simulink model "missileSystem"  (R2014a)
settings: Solver=ode45  StartTime=0.0  StopTime=10.0  MaxStep=0.2  RelTol=1e-3
values from neighbouring files (symbols this model uses):
  Arb = [A11 A12; A21 A22]    [getRigidBodySS.m]
  Brb = [B1;B2]    [getRigidBodySS.m]
  Crb = [Cx; CAccCG; CAcc]    [getRigidBodySS.m]
  Drb = [Dx; DAccCG; DAcc]    [getRigidBodySS.m]
  wF = 2*pi*50    (= 314.159265359)    [initMissilelFullIO.m]
  wT = 2*pi*25    (= 157.079632679)    [initMissilelFullIO.m]
  zF = 0.707    [initMissilelFullIO.m]
  zT = 0.707    [initMissilelFullIO.m]
libraries: RCTblocks x1
settings Model: Creator=s220385  LastModifiedBy=s220385
settings OptimizationCC: SimCompilerOptimization=off
settings DebuggingCC: MergeDetectMultiDrivingBlocksExec=error  FrameProcessingCompatibilityMsg=error
settings RTWCC: RTWCompilerOptimization=off

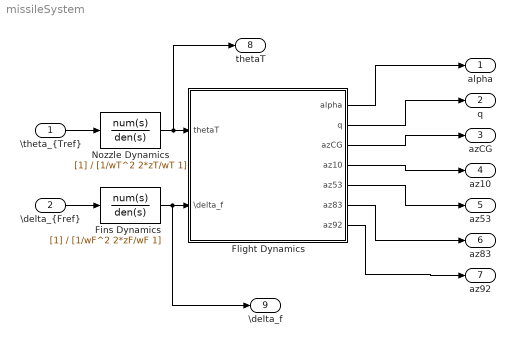
== system missileSystem ==
  "\\theta_{Tref}" : Inport
  "\\delta_{Fref}" : Inport  Port=2
  Fins Dynamics : TransferFcn  Denominator=[1/wF^2 2*zF/wF 1]
  Flight Dynamics : Subsystem  TreatAsAtomicUnit=on
      mask Display:
      | port_label('input', 1, '\theta_T','texmode','on')
      | port_label('input', 2, '\delta_F','texmode','on')
      | 
      | port_label('output', 1, '\alpha','texmode','on')
      | port_label('output', 2, 'q','texmode','on')
      | port_label('output', 3, 'a_{zCG}','texmode','on')
      | port_label('output', 4, 'a_{z10}','texmode','on')
      | port_label('output', 5, 'a_{z53}','texmode','on')
      | port_label('output', 6, 'a_{z83}','texmode','on')
      | port_label('output', 7, 'a_{z91}','texmode','on')
  Nozzle Dynamics : TransferFcn  Denominator=[1/wT^2 2*zT/wT 1]
  alpha : Outport
  q : Outport  Port=2
  azCG : Outport  Port=3
  az10 : Outport  Port=4
  az53 : Outport  Port=5
  az83 : Outport  Port=6
  az92 : Outport  Port=7
  "thetaT " : Outport  Port=8
  \delta_f : Outport  Port=9
  wires:
  Flight Dynamics/4(az10) -> az10/1
  Flight Dynamics/2(q) -> q/1
  Flight Dynamics/1(alpha) -> alpha/1
  "\\theta_{Tref}"/1 -> Nozzle Dynamics/1
  Flight Dynamics/3(azCG) -> azCG/1
  Flight Dynamics/5(az53) -> az53/1
  Flight Dynamics/6(az83) -> az83/1
  Flight Dynamics/7(az92) -> az92/1
  Nozzle Dynamics/1 -> "thetaT "/1, Flight Dynamics/1(thetaT)
  Fins Dynamics/1 -> \delta_f/1, Flight Dynamics/2(\delta_f)
  "\\delta_{Fref}"/1 -> Fins Dynamics/1

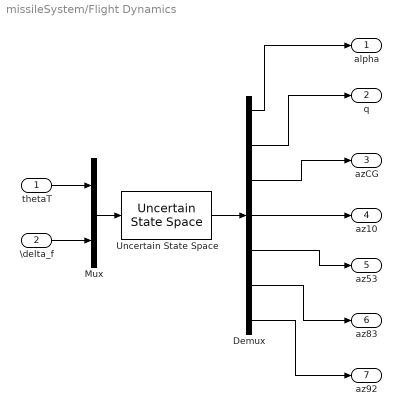
== system missileSystem/Flight Dynamics ==
  thetaT : Inport
  \delta_f : Inport  Port=2
  Demux : Demux  Outputs=7
  Mux : Mux  Inputs=2
  Uncertain State Space : RCTblocks/Uncertain State Space  Tag=USS  USystem=ss(Arb,Brb,Crb,Drb)  UValue=[]  X0=[]  uX0=[]
  alpha : Outport
  q : Outport  Port=2
  azCG : Outport  Port=3
  az10 : Outport  Port=4
  az53 : Outport  Port=5
  az83 : Outport  Port=6
  az92 : Outport  Port=7
  wires:
  Demux/3 -> azCG/1
  Demux/2 -> q/1
  Demux/4 -> az10/1
  Demux/1 -> alpha/1
  Demux/5 -> az53/1
  Demux/6 -> az83/1
  Demux/7 -> az92/1
  thetaT/1 -> Mux/1
  \delta_f/1 -> Mux/2
  Mux/1 -> Uncertain State Space/1
  Uncertain State Space/1 -> Demux/1
